simulink model "Supervisor_dados_reais_aceleracao"  (R2016a)
settings: Solver=VariableStepAuto  StartTime=0.0  StopTime=10.0  RelTol=1e-3
settings Model: Creator=vmaraccini-personal  LastModifiedBy=vmaraccini-personal
settings ModelReferenceCC: ModelReferenceNumInstancesAllowed=Single

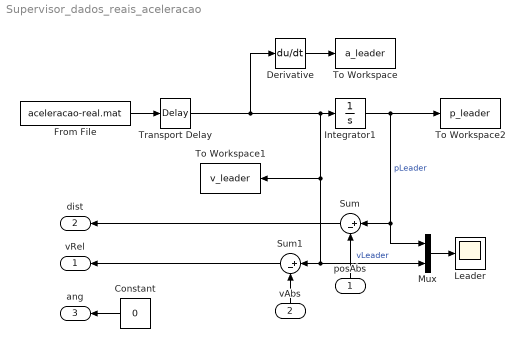
== system Supervisor_dados_reais_aceleracao ==
  posAbs : Inport
  vAbs : Inport  Port=2
  Constant : Constant  Value=0
  Derivative : Derivative
  From File : FromFile  FileName=aceleracao-real.mat  SampleTime=0
  Integrator1 : Integrator  InitialCondition=40
  Leader : Scope
  Mux : Mux  Inputs=2
  Sum : Sum  Inputs=|+-
  Sum1 : Sum  Inputs=|+-
  To Workspace : ToWorkspace  VariableName=a_leader  SampleTime=-1
      settings: Save2DSignal=2-D array (concatenate along first dimension)
  To Workspace1 : ToWorkspace  VariableName=v_leader  SampleTime=-1
      settings: Save2DSignal=2-D array (concatenate along first dimension)
  To Workspace2 : ToWorkspace  VariableName=p_leader  SampleTime=-1
      settings: Save2DSignal=2-D array (concatenate along first dimension)
  Transport Delay : TransportDelay  DelayTime=30  InitialOutput=13  TransDelayFeedthrough=on
  vRel : Outport
  dist : Outport  Port=2
  ang : Outport  Port=3
  wires:
  Integrator1/1 -> To Workspace2/1, Mux/1, Sum/1  "pLeader"
  Sum1/1 -> vRel/1
  vAbs/1 -> Sum1/2
  posAbs/1 -> Sum/2
  Sum/1 -> dist/1
  Transport Delay/1 -> Derivative/1, To Workspace1/1, Mux/2, Sum1/1, Integrator1/1  "vLeader"
  Constant/1 -> ang/1
  Derivative/1 -> To Workspace/1
  Mux/1 -> Leader/1
  From File/1 -> Transport Delay/1
